simulink model "RGR_Shendrikov_sim"  (R2020b)
settings: Solver=FixedStepDiscrete  StartTime=0.0  StopTime=10.0  RelTol=1e-3  EnableMultiTasking=on
values from neighbouring files (symbols this model uses):
  TaxRate = [0:0.05:0.75]    [RGR_Shendrikov.m]
undefined symbols (not defined in the file or in its folder): DiscIntNeverNeededParam, Profitability
settings Model: ExtModeTrigMode=oneshot  ExtModeArmWhenConnect=off  Creator=mluser  LastModifiedBy=mluser
settings DataIOCC: ExternalInput=Rntb  FinalStateName=BdjS  SaveFormat=Array  SignalLoggingSaveFormat=ModelDataLogs  SaveOutput=off  SaveTime=off  ReturnWorkspaceOutputs=off
settings OptimizationCC: BlockReduction=off  BooleanDataType=off  OptimizeBlockIOStorage=off
settings DebuggingCC: SaveWithParameterizedLinksMsg=none  UnderspecifiedInitializationDetection=Classic  MergeDetectMultiDrivingBlocksExec=none  SignalResolutionControl=TryResolveAllWithWarning  MultiTaskDSMMsg=warning  MultiTaskCondExecSysMsg=none
settings HardwareCC: TargetUnknown=on
settings ModelReferenceCC: PropagateSignalLabelsOutOfModel=off
settings GRTTargetCC: CombineOutputUpdateFcns=off  GRTInterface=on

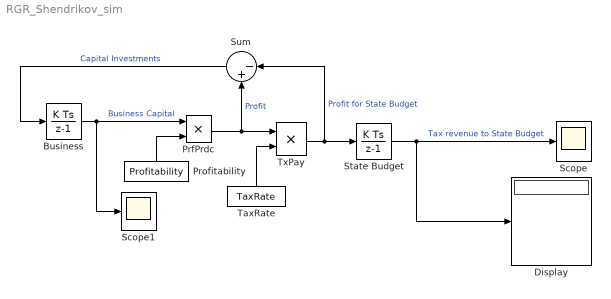
== system RGR_Shendrikov_sim ==
  Business : DiscreteIntegrator  InitialCondition=100  ICPrevOutput=DiscIntNeverNeededParam  ICPrevScaledInput=DiscIntNeverNeededParam
  Display : Display
  PrfPrdc : Product  SaturateOnIntegerOverflow=on
  Profitability : Constant  Value=Profitability
  Scope : Scope
  Scope1 : Scope
  State Budget : DiscreteIntegrator  ICPrevOutput=DiscIntNeverNeededParam  ICPrevScaledInput=DiscIntNeverNeededParam
  Sum : Sum  Inputs=|-+  SaturateOnIntegerOverflow=on
  TaxRate : Constant  Value=TaxRate
  TxPay : Product  SaturateOnIntegerOverflow=on
  wires:
  PrfPrdc/1 -> TxPay/1, Sum/2  "Profit"
  Sum/1 -> Business/1  "Capital Investments"
  TaxRate/1 -> TxPay/2
  TxPay/1 -> Sum/1, State Budget/1  "Profit for State Budget"
  Business/1 -> Scope1/1, PrfPrdc/1  "Business Capital"
  Profitability/1 -> PrfPrdc/2
  State Budget/1 -> Display/1, Scope/1  "Tax revenue to State Budget"
